simulink model "StateFlow_1"  (R2018a)
settings: Solver=VariableStepDiscrete  StartTime=0.0  StopTime=10  MaxStep=0.01  RelTol=1e-3
settings Model: PauseTimes=1  SnapshotBufferSize=2  SnapshotInterval=2  Creator=Choaib ELMADI  LastModifiedBy=Choaib ELMADI
settings HardwareCC: TargetBitPerPointer=64  TargetBitPerSizeT=64  TargetBitPerPtrDiffT=64  TargetLongLongMode=on  TargetIntDivRoundTo=Zero  TargetEndianess=LittleEndian  TargetWordSize=64  TargetHWDeviceType=MATLAB Host  ProdEqTarget=off
settings RTWCC: SystemTargetFile=rsim.tlc  TemplateMakefile=rsim_default_tmf  Description=Rapid Simulation Target  GenerateReport=on  LaunchReport=on
settings RSimTargetCC: TargetLangStandard=C99 (ISO)  GeneratePreprocessorConditionals=Use local settings

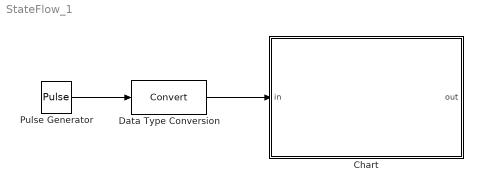
== system StateFlow_1 ==
  Chart : Stateflow chart  TreatAsAtomicUnit=on
  Data Type Conversion : DataTypeConversion
  Pulse Generator : DiscretePulseGenerator  PulseType=Time based  Period=3  PulseWidth=50
  wires:
  Pulse Generator/1 -> Data Type Conversion/1
  Data Type Conversion/1 -> Chart/1(in)

== stateflow chart StateFlow_1/Chart ==
  state ON_STATE
    out = 1
    local_data = 10
  state OFF_STATE
    out = 0
    local_data = 20
  (default) -> ON_STATE
  ON_STATE -> OFF_STATE : [in==0]
  OFF_STATE -> ON_STATE : [in==1]
  data: out output int8; in input int8; local_data local double [10..100] =15
